simulink model "tutorial12_kalman"  (R2025a)
settings: Solver=VariableStepAuto  StartTime=0.0  StopTime=5  RelTol=1e-3
libraries: simulink x2
settings Model: Creator=xing2  LastModifiedBy=xing2

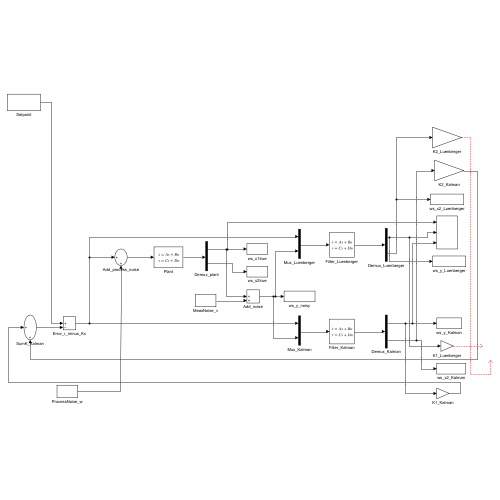
[thumbnail: Simulink's stored preview of the top-level diagram]
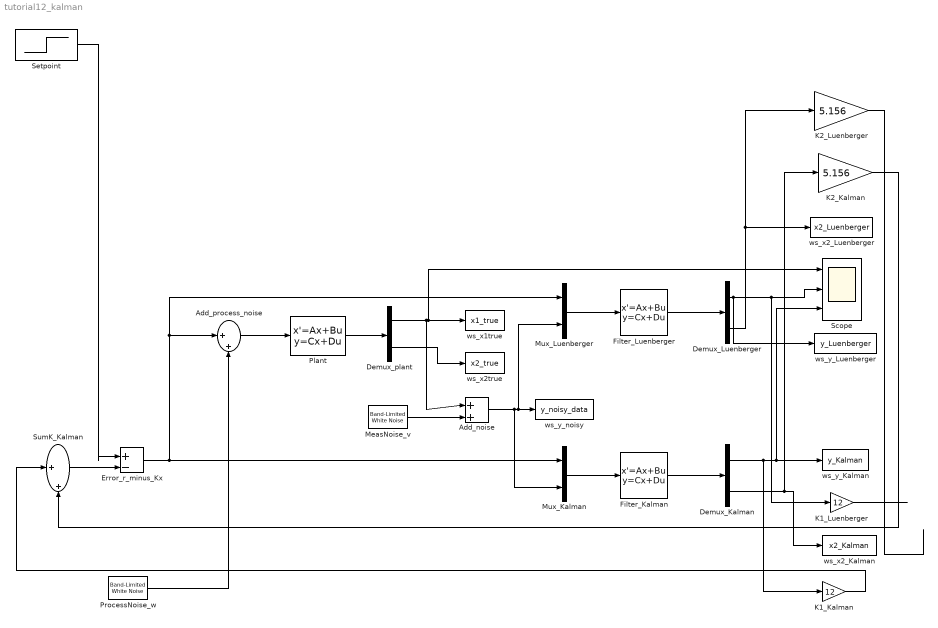
== system tutorial12_kalman ==
  Add_noise : Sum  Inputs=|++
  Add_process_noise : Sum  Inputs=|++
  Demux_Kalman : Demux  Outputs=2
  Demux_Luenberger : Demux  Outputs=2
  Demux_plant : Demux  Outputs=2
  Error_r_minus_Kx : Sum  Inputs=|+-
  Filter_Kalman : StateSpace  A=[-2.86892696129517 1;-6.11537095462317 -0.5]  B=[0 2.86892696129517;1 2.11537095462317]  C=[1 0;0 1]  D=[0 0;0 0]  InitialCondition=[0; 0]
  Filter_Luenberger : StateSpace  A=[-13.5 1;-41.2499999999999 -0.5]  B=[0 13.5;1 37.2499999999999]  C=[1 0;0 1]  D=[0 0;0 0]  InitialCondition=[0; 0]
  K1_Kalman : Gain  Gain=12
  K1_Luenberger : Gain  Gain=12
  K2_Kalman : Gain  Gain=5.156
  K2_Luenberger : Gain  Gain=5.156
  MeasNoise_v : simulink/Sources/Band-Limited White Noise  Cov=[0.1]  Ts=0.1  seed=[23341]
  Mux_Kalman : Mux  Inputs=2
  Mux_Luenberger : Mux  Inputs=2
  Plant : StateSpace  A=[0 1;-4 -0.5]  B=[0;1]  C=eye(2)  D=zeros(2,1)  InitialCondition=[0.2; 0]
  ProcessNoise_w : simulink/Sources/Band-Limited White Noise  Cov=[0.1]  Ts=0.1  seed=[23341]
  Scope : Scope  NumInputPorts=3
  Setpoint : Step  Time=0.5  SampleTime=0
  SumK_Kalman : Sum  Inputs=|++
  ws_x1true : ToWorkspace  VariableName=x1_true  SaveFormat=Timeseries  SampleTime=-1
  ws_x2_Kalman : ToWorkspace  VariableName=x2_Kalman  SaveFormat=Timeseries  SampleTime=-1
  ws_x2_Luenberger : ToWorkspace  VariableName=x2_Luenberger  SaveFormat=Timeseries  SampleTime=-1
  ws_x2true : ToWorkspace  VariableName=x2_true  SaveFormat=Timeseries  SampleTime=-1
  ws_y_Kalman : ToWorkspace  VariableName=y_Kalman  SaveFormat=Timeseries  SampleTime=-1
  ws_y_Luenberger : ToWorkspace  VariableName=y_Luenberger  SaveFormat=Timeseries  SampleTime=-1
  ws_y_noisy : ToWorkspace  VariableName=y_noisy_data  SaveFormat=Timeseries  SampleTime=-1
  wires:
  Plant/1 -> Demux_plant/1
  Setpoint/1 -> Error_r_minus_Kx/1
  SumK_Kalman/1 -> Error_r_minus_Kx/2
  Filter_Kalman/1 -> Demux_Kalman/1
  Error_r_minus_Kx/1 -> Mux_Luenberger/1, Add_process_noise/1, Mux_Kalman/1
  Demux_plant/1 -> Scope/1, ws_x1true/1, Add_noise/1
  K1_Luenberger/1 -> ?
  ProcessNoise_w/1 -> Add_process_noise/2
  Add_process_noise/1 -> Plant/1
  Filter_Luenberger/1 -> Demux_Luenberger/1
  Demux_plant/2 -> ws_x2true/1
  Mux_Luenberger/1 -> Filter_Luenberger/1
  MeasNoise_v/1 -> Add_noise/2
  Add_noise/1 -> Mux_Luenberger/2, ws_y_noisy/1, Mux_Kalman/2
  Demux_Luenberger/2 -> K2_Luenberger/1, ws_x2_Luenberger/1
  Mux_Kalman/1 -> Filter_Kalman/1
  Demux_Luenberger/1 -> Scope/2, K1_Luenberger/1, ws_y_Luenberger/1
  Demux_Kalman/1 -> Scope/3, ws_y_Kalman/1, K1_Kalman/1
  Demux_Kalman/2 -> K2_Kalman/1, ws_x2_Kalman/1
  K2_Luenberger/1 -> ?
  K2_Kalman/1 -> SumK_Kalman/2
  K1_Kalman/1 -> SumK_Kalman/1
